simulink model "Traffic_Light"  (R2020b)
settings: Solver=VariableStepAuto  StartTime=0.0  StopTime=200  RelTol=1e-3
undefined symbols (not defined in the file): DiscIntNeverNeededParam
libraries: simulink x1
settings Model: Creator=vijay jagtap  LastModifiedBy=vijay jagtap

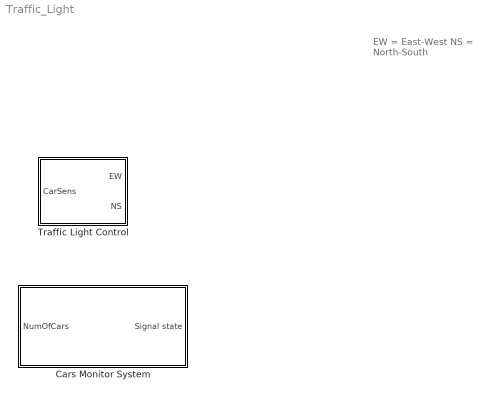
== system Traffic_Light ==
  note: EW = East-West
      | NS = North-South
  Cars Monitor System : Subsystem
  Traffic Light Control : Stateflow chart  TreatAsAtomicUnit=on

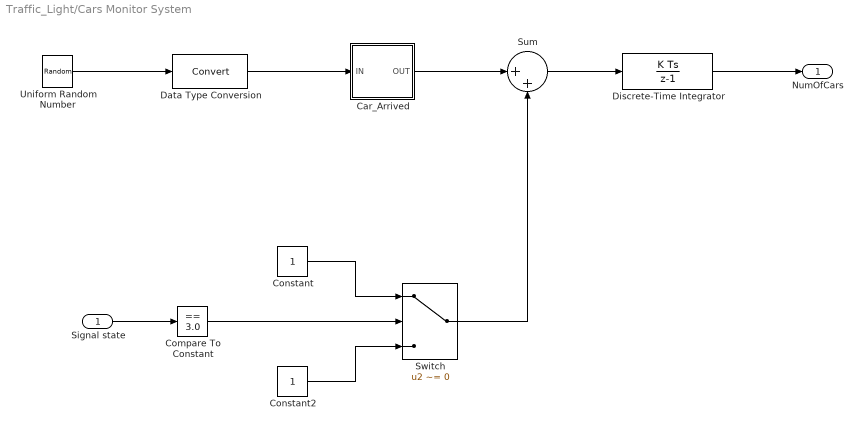
== system Traffic_Light/Cars Monitor System ==
  Signal state : Inport
  Car_Arrived : Stateflow chart  TreatAsAtomicUnit=on
  Compare To Constant : simulink/Logic and Bit Operations/Compare To Constant  relop===  const=3.0  OutDataTypeStr=boolean
  Constant : Constant
  Constant2 : Constant
  Data Type Conversion : DataTypeConversion
  Discrete-Time Integrator : DiscreteIntegrator  SampleTime=-1  LimitOutput=on  LowerSaturationLimit=0  ICPrevOutput=DiscIntNeverNeededParam  ICPrevScaledInput=DiscIntNeverNeededParam
  Sum : Sum  Inputs=|++
  Switch : Switch  Criteria=u2 ~= 0
  Uniform Random Number : UniformRandomNumber  Minimum=0  Maximum=100  SampleTime=0
  NumOfCars : Outport
  wires:
  Uniform Random Number/1 -> Data Type Conversion/1
  Data Type Conversion/1 -> Car_Arrived/1(IN)
  Car_Arrived/1(OUT) -> Sum/1
  Sum/1 -> Discrete-Time Integrator/1
  Compare To Constant/1 -> Switch/2
  Constant/1 -> Switch/1
  Constant2/1 -> Switch/3
  Signal state/1 -> Compare To Constant/1
  Switch/1 -> Sum/2
  Discrete-Time Integrator/1 -> NumOfCars/1

== stateflow chart Traffic_Light/Cars Monitor System/Car_Arrived ==
  (default) -> (junction 1) : {OUT = IN > 90;}
  data: IN input; OUT output

== stateflow chart Traffic_Light/Traffic Light Control ==
  state STOP
    NS = RED;
    EW = GREEN;
  state StopForTraffic
    NS = RED;
    EW = GREEN;
  state WaitToGo
    NS = RED;
    EW = YELLOW;
  state Go
    NS = GREEN;
    EW = RED;
  state GoToStop
    NS = YELLOW;
    EW = RED;
  (default) -> STOP
  STOP -> StopForTraffic : after(20,tick)
  StopForTraffic -> WaitToGo : [CarSens]
  WaitToGo -> Go : after(3,tick)
  Go -> GoToStop : after(10,tick)
  GoToStop -> STOP : after(3,tick)
  data: YELLOW constant double =2; GREEN constant double =3; RED constant double =1; CarSens input; EW output; NS output
